simulink subsystem "State_Machine_S2"  (R2023b)
settings: Solver=VariableStepAuto  StartTime=0.0  StopTime=10.0  RelTol=1e-3
settings Model: Creator=Inver  LastModifiedBy=Inver

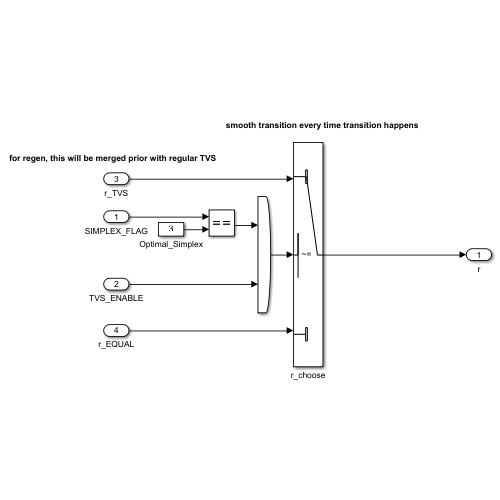
[thumbnail: Simulink's stored preview of the top-level diagram]
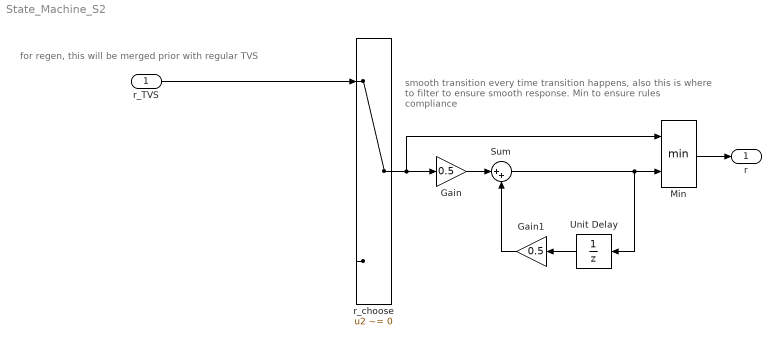
== system State_Machine_S2 ==
  note: for regen, this will be merged prior with regular TVS
  note: smooth transition every time transition happens, also this is where to filter to ensure smooth response. Min to ensure rules compliance
  r_TVS : Inport
  Gain : Gain  Gain=0.5
  Gain1 : Gain  Gain=0.5
  Min : MinMax  Inputs=2
  Sum : Sum  Inputs=|++
  Unit Delay : UnitDelay  SampleTime=-1  HasFrameUpgradeWarning=on
  r_choose : Switch  Criteria=u2 ~= 0  OutDataTypeStr=double  SaturateOnIntegerOverflow=off  InputSameDT=off
  r : Outport
  wires:
  r_choose/1 -> Gain/1, Min/1
  r_TVS/1 -> r_choose/1
  Sum/1 -> Unit Delay/1, Min/2
  Gain/1 -> Sum/1
  Unit Delay/1 -> Gain1/1
  Gain1/1 -> Sum/2
  Min/1 -> r/1
